simulink model "simulator"  (R2024b)
settings: Solver=VariableStepAuto  StartTime=0.0  StopTime=20  RelTol=1e-3
values from neighbouring files (symbols this model uses):
  dot_elev_0 = deg2rad(0)    [simulation_params.m]
  dot_pitch_0 = deg2rad(0)    [simulation_params.m]
  dot_trav_0 = deg2rad(0)    [simulation_params.m]
  elev_0 = deg2rad(-30)    [simulation_params.m]
  elev_max = deg2rad(30)    [HeliSystem.m]    (also in simulation_params.m)
  elev_min = deg2rad(-30)    [HeliSystem.m]    (also in simulation_params.m)
  pitch_0 = deg2rad(0)    [simulation_params.m]
  pitch_max = deg2rad(90)    [HeliSystem.m]    (also in simulation_params.m)
  pitch_min = deg2rad(-90)    [HeliSystem.m]    (also in simulation_params.m)
  trav_0 = deg2rad(0)    [simulation_params.m]
  trav_max = deg2rad(180)    [HeliSystem.m]    (also in simulation_params.m)
  trav_min = deg2rad(-180)    [HeliSystem.m]    (also in simulation_params.m)
settings Model: Creator=bryankikuta  LastModifiedBy=bryankikuta

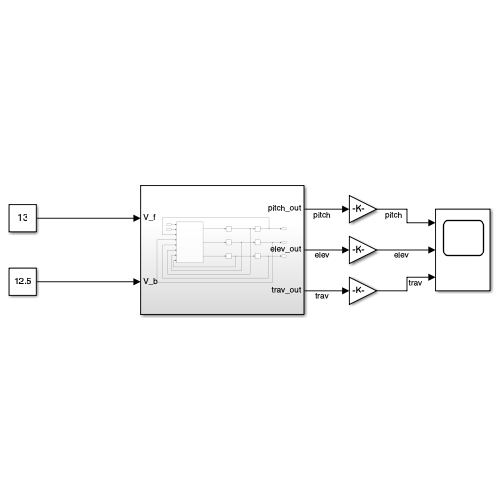
[thumbnail: Simulink's stored preview of the top-level diagram]
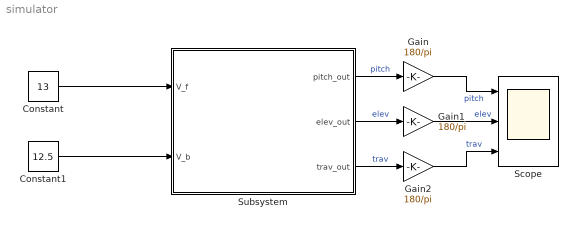
== system simulator ==
  Constant : Constant  Value=13
  Constant1 : Constant  Value=12.5
  Gain : Gain  Gain=180/pi
  Gain1 : Gain  Gain=180/pi
  Gain2 : Gain  Gain=180/pi
  Scope : Scope  NumInputPorts=3
  Subsystem : Subsystem
  wires:
  Constant/1 -> Subsystem/1(V_f)
  Subsystem/2(elev_out) -> Gain1/1  "elev"
  Subsystem/1(pitch_out) -> Gain/1  "pitch"
  Subsystem/3(trav_out) -> Gain2/1  "trav"
  Gain/1 -> Scope/1  "pitch"
  Gain1/1 -> Scope/2  "elev"
  Gain2/1 -> Scope/3  "trav"
  Constant1/1 -> Subsystem/2(V_b)

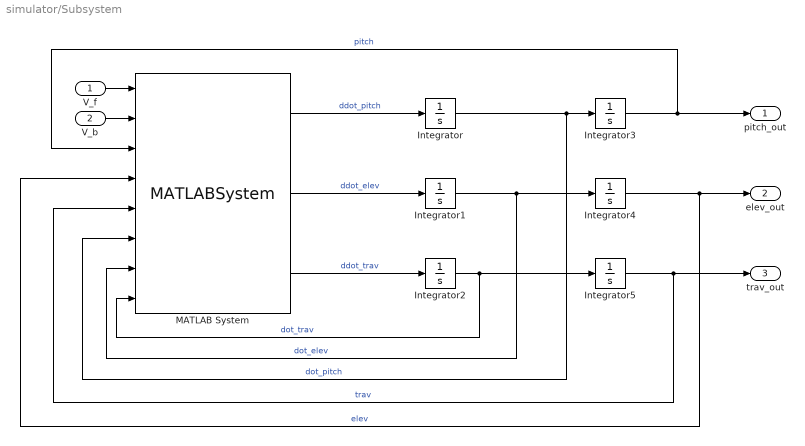
== system simulator/Subsystem ==
  V_f : Inport
  V_b : Inport  Port=2
  Integrator : Integrator  InitialCondition=dot_pitch_0
  Integrator1 : Integrator  InitialCondition=dot_elev_0
  Integrator2 : Integrator  InitialCondition=dot_trav_0
  Integrator3 : Integrator  InitialCondition=pitch_0  LimitOutput=on  UpperSaturationLimit=pitch_max  LowerSaturationLimit=pitch_min
  Integrator4 : Integrator  InitialCondition=elev_0  LimitOutput=on  UpperSaturationLimit=elev_max  LowerSaturationLimit=elev_min
  Integrator5 : Integrator  InitialCondition=trav_0  LimitOutput=on  UpperSaturationLimit=trav_max  LowerSaturationLimit=trav_min
  MATLAB System : MATLABSystem  System=HeliSystem  V_max=30  a_thrust=0.0053  b_thrust=0.0022  a_torque=0.0003  b_torque=0.0004  b_1=0.20  b_2=0.238  b_3=25.75 * 0.0254  b_4=0.0513  L_h=6.985 * 0.0254  L_a=25.75 * 0.0254  L_w=18.125 * 0.0254  g=9.81  T_stat_pitch=0.001  T_stat_elev=0.001  T_stat_trav=0.005  T_coeff_pitch=0.1  T_coeff_elev=0.1  T_coeff_trav=0.1  m_f=0.721  m_b=0.721  m_w=1.914  ax_pitch=[ 1; 0; 0 ]  ax_elev=[ 0; 1; 0 ]  ax_trav=[ 0; 0; 1 ]  F_f=[ 0; 0; -1 ]  F_b=[ 0; 0; -1 ]  T_f=[ 0; 0; 1 ]  T_b=[ 0; 0; -1 ]  SimulateUsing=Code generation
      mask Type: HeliSystem
      mask Display:
      | disp('HeliSystem');
      | port_label('input',1,'V_f');
      | port_label('input',2,'V_b');
      | port_label('input',3,'pitch');
      | port_label('input',4,'elev');
      | port_label('input',5,'trav');
      | port_label('input',6,'dot_pitch');
      | port_label('input',7,'dot_elev');
      | port_label('input',8,'dot_trav');
      | port_label('output',1,'ddot_pitch');
      | port_label('output',2,'ddot_elev');
      | port_label('output',3,'ddot_trav');
  pitch_out : Outport
  elev_out : Outport  Port=2
  trav_out : Outport  Port=3
  wires:
  V_b/1 -> MATLAB System/2
  Integrator4/1 -> MATLAB System/4, elev_out/1  "elev"
  MATLAB System/2 -> Integrator1/1  "ddot_elev"
  Integrator5/1 -> MATLAB System/5, trav_out/1  "trav"
  Integrator/1 -> MATLAB System/6, Integrator3/1  "dot_pitch"
  V_f/1 -> MATLAB System/1
  Integrator2/1 -> MATLAB System/8, Integrator5/1  "dot_trav"
  MATLAB System/3 -> Integrator2/1  "ddot_trav"
  MATLAB System/1 -> Integrator/1  "ddot_pitch"
  Integrator1/1 -> MATLAB System/7, Integrator4/1  "dot_elev"
  Integrator3/1 -> MATLAB System/3, pitch_out/1  "pitch"
